simulink library "test_px4"  (R2022b)
settings: Solver=VariableStepAuto  StartTime=0.0  StopTime=10.0  RelTol=1e-3
libraries: uavmavlinklib x2, dspnetwork x2, shared6dof x1
settings Model: Creator=User  LastModifiedBy=User

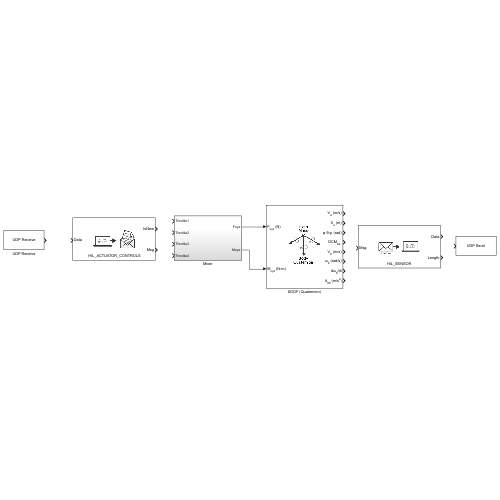
[thumbnail: Simulink's stored preview of the top-level diagram]
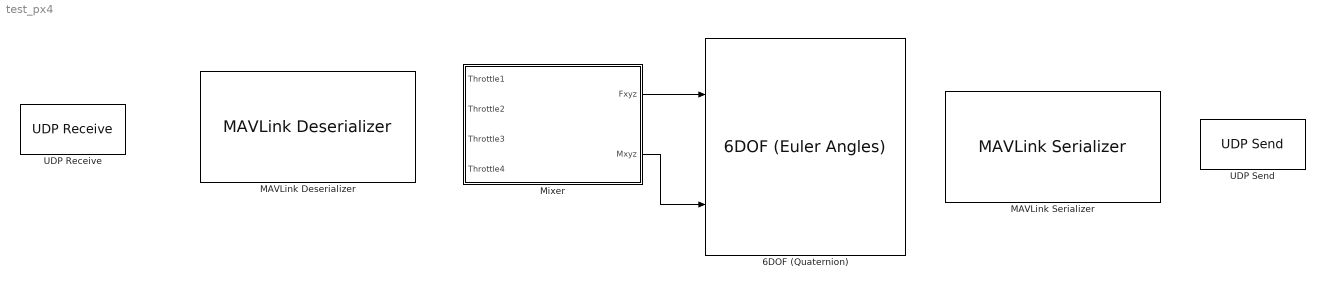
== system test_px4 ==
  6DOF (Quaternion) : shared6dof/6DOF (Euler Angles)  units=Metric (MKS)  mtype=Fixed  rep=Quaternion  xme_0=[0 0 0]  Vm_0=[0 0 0]  eul_0=[0 0 0]  pm_0=[0 0 0]  mass_0=1.0  mass_e=0.5  mass_f=2.0  inertia=eye(3)  inertia_e=eye(3)  inertia_f=2*eye(3)  k_quat=1.0  vre_flag=on  abi_flag=off  aMode=0  xme_statename=''  Vm_statename=''  eul_statename=''  quat_statename=''  pm_statename=''  mass_statename=''
      settings: LibrarySourceBlock=aerolib6dof2/6DOF (Quaternion)
  MAVLink Deserializer : uavmavlinklib/MAVLink Deserializer  dialectSource=Select from standard MAVLink dialects  dialect=common.xml  dialectCustom=common.xml  version=2  messageType=HIL_ACTUATOR_CONTROLS  inputDataLength=off  SystemIDFilter=off  systemID=1  ComponentIDFilter=off  componentID=1  queueMsg=off  queueMsgSize=50  dropNum=off
  MAVLink Serializer : uavmavlinklib/MAVLink Serializer  dialectSource=Select from standard MAVLink dialects  dialect=common.xml  dialectCustom=common.xml  version=2  messageType=HIL_SENSOR
  Mixer : Subsystem
  UDP Receive : dspnetwork/UDP Receive  localURL='0.0.0.0'  localPort=25000  remoteURL='0.0.0.0'  remotePort=-1  recvBufferSize=8192  dims=255  signalDatatype=uint8  isComplex=off  isVarSize=on  showBlockingTime=off  blockingTime=0  sampletime=1  blockPlatform=[]
      settings: LibrarySourceBlock=dspsrcs4/UDP Receive
  UDP Send : dspnetwork/UDP Send  remoteURL='127.0.0.1'  remotePort=25000  localURL='0.0.0.0'  localPortSource=Automatically determine  localPort=-1  sendBufferSize=8192  sampletime=-1  blockPlatform=[]  separateLengthPort=0
      settings: LibrarySourceBlock=dspsnks4/UDP Send
  wires:
  Mixer/1(Fxyz) -> 6DOF (Quaternion)/1
  Mixer/2(Mxyz) -> 6DOF (Quaternion)/2

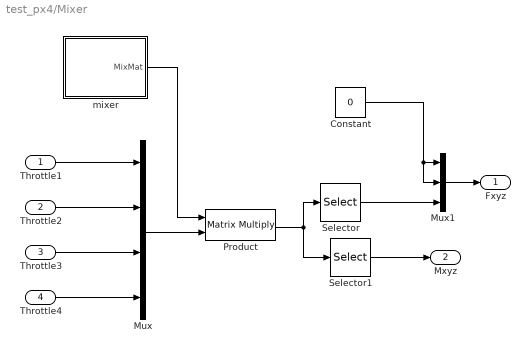
== system test_px4/Mixer ==
  Throttle1 : Inport
  Throttle2 : Inport  Port=2
  Throttle3 : Inport  Port=3
  Throttle4 : Inport  Port=4
  Constant : Constant  Value=0
  Mux : Mux
  Mux1 : Mux  Inputs=3
  Product : Product  Multiplication=Matrix(*)
  Selector : Selector  InputPortWidth=4  IndexOptions=Index vector (dialog)  Indices=[1]  OutputSizes=1
  Selector1 : Selector  InputPortWidth=4  IndexOptions=Index vector (dialog)  Indices=[2 3 4]  OutputSizes=1
  mixer : Subsystem
  Fxyz : Outport
  Mxyz : Outport  Port=2
  wires:
  Throttle1/1 -> Mux/1
  Throttle4/1 -> Mux/4
  Throttle3/1 -> Mux/3
  Throttle2/1 -> Mux/2
  Mux/1 -> Product/2
  mixer/1(MixMat) -> Product/1
  Product/1 -> Selector/1, Selector1/1
  Selector1/1 -> Mxyz/1
  Mux1/1 -> Fxyz/1
  Constant/1 -> Mux1/2, Mux1/1
  Selector/1 -> Mux1/3

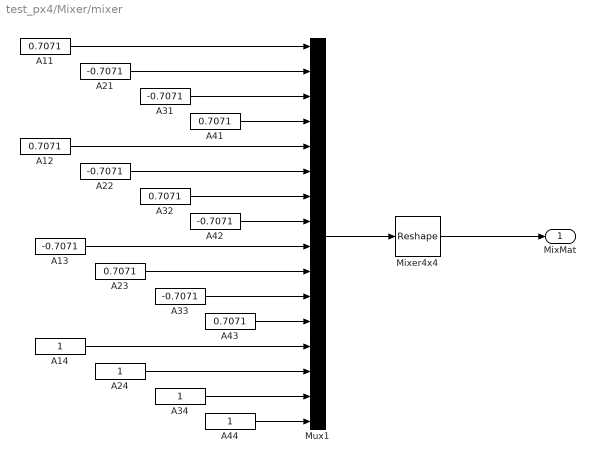
== system test_px4/Mixer/mixer ==
  A{11..12,23,32,41,43} (6 alike) : Constant  Value=0.7071
  A{13,21..22,31,33,42} (6 alike) : Constant  Value=-0.7071
  A{14,24,34,44} (4 alike) : Constant
  Mixer4x4 : Reshape  OutputDimensionality=Customize  OutputDimensions=[4,4]
  Mux1 : Mux  Inputs=16
  MixMat : Outport
  wires:
  A11/1 -> Mux1/1
  Mux1/1 -> Mixer4x4/1
  Mixer4x4/1 -> MixMat/1
  A21/1 -> Mux1/2
  A31/1 -> Mux1/3
  A41/1 -> Mux1/4
  A32/1 -> Mux1/7
  A12/1 -> Mux1/5
  A22/1 -> Mux1/6
  A42/1 -> Mux1/8
  A23/1 -> Mux1/10
  A33/1 -> Mux1/11
  A13/1 -> Mux1/9
  A43/1 -> Mux1/12
  A34/1 -> Mux1/15
  A24/1 -> Mux1/14
  A14/1 -> Mux1/13
  A44/1 -> Mux1/16
